simulink model "Synch_Gen2"  (Simulink 4.00)
settings: Solver=ode23tb  StartTime=0.0  StopTime=5
InitFcn:
  | powericon('psbinitsys',bdroot);
libraries: powerlib2 x8, powerlib_extras x5
settings Model: LastModifiedBy=ieao  SaveTime=off  SaveOutput=off  LimitDataPoints=off  BlockReductionOpt=off

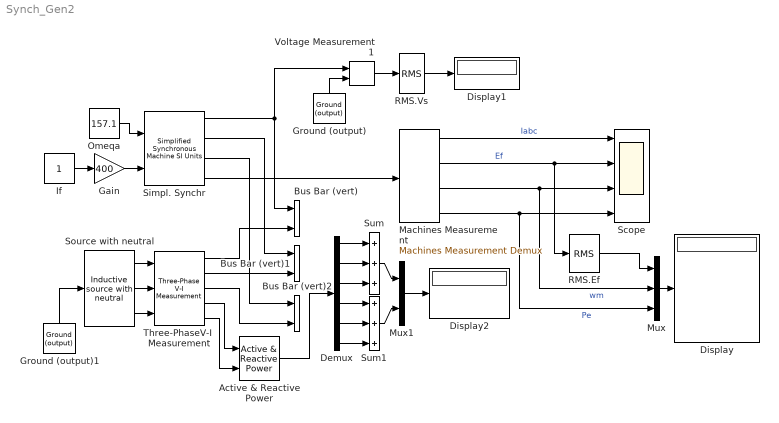
== system Synch_Gen2 ==
  Active & Reactive Power : powerlib_extras/Measurements/Active & Reactive Power  f1=60
  Bus Bar (vert) : powerlib2/Connectors/Bus Bar (vert)  Tag=PoWeRsYsTeMbLoCk  entrees=2  sorties=0  PSBOutputType=11111111111111111111111111111111111111111111111111111111111111111111111111111111111111111
  Bus Bar (vert)1 : powerlib2/Connectors/Bus Bar (vert)  Tag=PoWeRsYsTeMbLoCk  entrees=2  sorties=0  PSBOutputType=11111111111111111111111111111111111111111111111111111111111111111111111111111111111111111
  Bus Bar (vert)2 : powerlib2/Connectors/Bus Bar (vert)  Tag=PoWeRsYsTeMbLoCk  entrees=2  sorties=0  PSBOutputType=11111111111111111111111111111111111111111111111111111111111111111111111111111111111111111
  Demux : Demux  Outputs=6  BusSelectionMode=off
  Display : Display
      settings: Format=short
  Display1 : Display
      settings: Format=short  SampleTime=0
  Display2 : Display
      settings: Format=short  SampleTime=0.02
  Gain : Gain  Gain=400  Multiplication=Element-wise(K.*u)  SaturateOnIntegerOverflow=on
  Ground (output) : powerlib2/Connectors/Ground (output)  Tag=PoWeRsYsTeMbLoCk  Orientation=up  PSBOutputType=1
  Ground (output)1 : powerlib2/Connectors/Ground (output)  Tag=PoWeRsYsTeMbLoCk  Orientation=up  PSBOutputType=1
  If : Constant  Value=1
  Machines Measurement : powerlib2/Machines/Machines Measurement Demux  machType=Simplified synchronous  ssm1=on  ssm2=off  ssm3=on  ssm4=off  ssm5=on  ssm6=on  sm1=on  sm2=off  sm3=on  sm4=off  sm5=off  sm6=off  sm7=off  sm8=on  sm9=on  sm10=off  sm11=off  asm1=on  asm2=on  asm3=on  asm4=on  asm5=on  asm6=on  asm7=on  asm8=on  asm9=on  asm10=on  asm11=on  pmsm1=on  pmsm2=on  pmsm3=on  pmsm4=on  pmsm5=on  pmsm6=on  lastType=1
  Mux : Mux  Inputs=3
  Mux1 : Mux  Inputs=2
  Omeqa : Constant  Value=157.1
  RMS.Ef : powerlib_extras/Measurements/RMS  f1=50
  RMS.Vs : powerlib_extras/Measurements/RMS  f1=50
  Scope : Scope  NumInputPorts=4
      settings: TimeRange=auto  YMin=-500~-500~149.226~0  YMax=400~500~164.934~15000  SaveToWorkspace=off  SaveName=ScopeData  MaxDataPoints=5000
  "Simpl. Synchr " : powerlib2/Machines/Simplified Synchronous  Machine SI Units  Tag=PoWeRsYsTeMbLoCk  conType=3-wire Y  x1=[ 100e3,380,50 ]  x2=[ inf,0,2 ]  x3=[ 0. 0.9e-3 ]  x4="[ 0   0   0,0,0   0,0,0 ]"  PSBOutputType=1111  iounits=1
  Source with neutral : powerlib_extras/Three-Phase Library/Inductive source with neutral  V=310  Phi=0  F=50  R=0.001  L=0
  Sum : Sum  Inputs=+++  SaturateOnIntegerOverflow=on
  Sum1 : Sum  Inputs=+++  SaturateOnIntegerOverflow=on
  Three-PhaseV-I  Measurement : powerlib_extras/Measurements/Three-Phase V-I Measurement  phaseurs=off  Vpu=off  Vbase=500e3  Ppu=off  Pbase=100e6
  Voltage Measurement1 : powerlib2/Measurements/Voltage Measurement  Tag=PoWeRsYsTeMmEaSuReMeNt  PSBOutputType=0  PSBequivalent=1
  wires:
  "Simpl. Synchr "/1 -> Voltage Measurement1/1, Bus Bar (vert)/1
  "Simpl. Synchr "/2 -> Bus Bar (vert)1/1
  "Simpl. Synchr "/3 -> Bus Bar (vert)2/1
  "Simpl. Synchr "/4 -> Machines Measurement/1
  Omeqa/1 -> "Simpl. Synchr "/1
  Machines Measurement/1 -> Scope/1  "Iabc"
  Voltage Measurement1/1 -> RMS.Vs/1
  RMS.Vs/1 -> Display1/1
  Ground (output)/1 -> Voltage Measurement1/2
  Machines Measurement/2 -> Scope/2, RMS.Ef/1  "Ef"
  Machines Measurement/3 -> Scope/3, Mux/2  "wm"
  Machines Measurement/4 -> Scope/4, Mux/3  "Pe"
  RMS.Ef/1 -> Mux/1
  Mux/1 -> Display/1
  Three-PhaseV-I  Measurement/3 -> Bus Bar (vert)2/2
  Source with neutral/1 -> Three-PhaseV-I  Measurement/1
  Source with neutral/2 -> Three-PhaseV-I  Measurement/2
  Source with neutral/3 -> Three-PhaseV-I  Measurement/3
  Active & Reactive Power/1 -> Demux/1
  Three-PhaseV-I  Measurement/1 -> Bus Bar (vert)/2
  Three-PhaseV-I  Measurement/2 -> Bus Bar (vert)1/2
  Three-PhaseV-I  Measurement/4 -> Active & Reactive Power/1
  Three-PhaseV-I  Measurement/5 -> Active & Reactive Power/2
  Demux/1 -> Sum/1
  Demux/2 -> Sum/2
  Demux/3 -> Sum/3
  Demux/4 -> Sum1/1
  Demux/5 -> Sum1/2
  Demux/6 -> Sum1/3
  Sum/1 -> Mux1/1
  Sum1/1 -> Mux1/2
  Mux1/1 -> Display2/1
  Gain/1 -> "Simpl. Synchr "/2
  If/1 -> Gain/1
  Ground (output)1/1 -> Source with neutral/1
